simulink model "sm_3d_printer"  (R2022a)
settings: Solver=FixedStepAuto  StartTime=0.0  StopTime=inf  FixedStep=0.005  RelTol=1e-3
model workspace: external: MATLAB File sm_3d_printer_parameters.m (data not in the file)
undefined symbols (not defined in the file): smiData, X, Y, Z
libraries: sm_lib x33, fl_lib x15, nesl_utility x10, ee_lib x3, slpidlib x3
(part 1 of 3)
settings Model: PacingRate=0.250000  Creator=The MathWorks, Inc.  LastModifiedBy=ale
settings SolverCC: AlgebraicLoopSolver=TrustRegion
settings DataIOCC: ReturnWorkspaceOutputs=off  SignalLoggingName=logsout_sm_3d_printer  ReturnWorkspaceOutputsName=tp3277b97d_6d31_4550_b739_ddfa201eda0b
settings DebuggingCC: UnconnectedInputMsg=warning  UnconnectedOutputMsg=warning  UnconnectedLineMsg=warning  SFMachineParentedDataDiag=warning
settings RTWCC: DLArmComputeVersion=19.05
settings SimscapeCC: SimscapeLogType=all  SimscapeLogSimulationStatistics=on  SimscapeLogName=simlog_sm_3d_printer  SimscapeLogLimitData=off  SimscapeLogDataHistory=6000
settings ExplorerConfigSet: InternalSimMechanicsExplorerSettings="<ExplorerConfiguration><canonicalview>default</canonicalview><AnimationSetting><BasePlaybackSpeed>1.0</BasePlaybackSpeed><PlaybackSpeedFactor>1.0</PlaybackSpeedFactor></AnimationSetting><TilePanel><TileInfo><Tiles Columns=\"2\" Count=\"3\" Rows=\"2\"><Column Weight=\"0.4991\"/><Column Weight=\"0.5009\"/><Row Weight=\"0.5\"/><Row Weight=\"0.5\"/><Tile Height=\"2\" Width=\"1\" X=\"0\" Y=\"0\"/><Tile Height=\"1\" Width=\"1\" X=\"1\" Y=\"0\"/><Tile Height=\"1\" Width=\"1\" X=\"1\" Y=\"1\"/></Tiles></TileInfo><SceneInfo><SceneViewer><BGColor><R>1</R><G>1</G><B>1</B></BGColor><Camera><DoPerspective>off</DoPerspective><Position><X>0.517183646619549187</X><Y>-0.517183616511187494</Y><Z>0.756683602090616692</Z></Position><Center><X>-0.0601666225700767041</X><Y>0.0601666526784384315</Y><Z>0.179333332900990905</Z></Center><Up><X>-0.408248290463863073</X><Y>0.408248290463863073</Y><Z>0.816496580927726145</Z></Up><ViewLimDist>1</ViewLimDist><YLim>0.950683694503029364</YLim><XLim>0.650749683842918647</XLim></Camera></SceneViewer><SceneViewer><BGColor><R>1</R><G>1</G><B>1</B></BGColor><Camera><DoPerspective>off</DoPerspective><Position><X>-0.0490736034624795273</X><Y>-0.0707121472427751085</Y><Z>1.81681125048728176</Z></Position><Center><X>-0.0490736034624795273</X><Y>-0.0707121472427751085</Y><Z>0.388900037674711374</Z></Center><Up><X>0</X><Y>1</Y><Z>-0</Z></Up><ViewLimDist>1</ViewLimDist><YLim>0.613605105866690814</YLim><XLim>0.865431478794638998</XLim></Camera></SceneViewer><SceneViewer><BGColor><R>1</R><G>1</G><B>1</B></BGColor><Camera><DoPerspective>off</DoPerspective><Position><X>-0.0653022372858333144</X><Y>-1.68343497325259128</Y><Z>0.329149100724004773</Z></Position><Center><X>-0.0653022372858333144</X><Y>-0.0588999497118882775</Y><Z>0.329149100724004773</Z></Center><Up><X>0</X><Y>-0</Y><Z>1</Z></Up><ViewLimDist>1</ViewLimDist><YLim>0.614884320576226218</YLim><XLim>0.867235689136411469</XLim></Camera></SceneViewer></SceneInfo></TilePanel><MechEditorPanel><Cameras/><GfxPanelCameraMap/><VideoCreator><PlaybackSpeedRatio>1.0</PlaybackSpeedRatio><FrameRate>30</FrameRate><VideoFormat>Motion JPEG AVI</VideoFormat><FrameSize>auto</FrameSize></VideoCreator></MechEditorPanel></ExplorerConfiguration>"

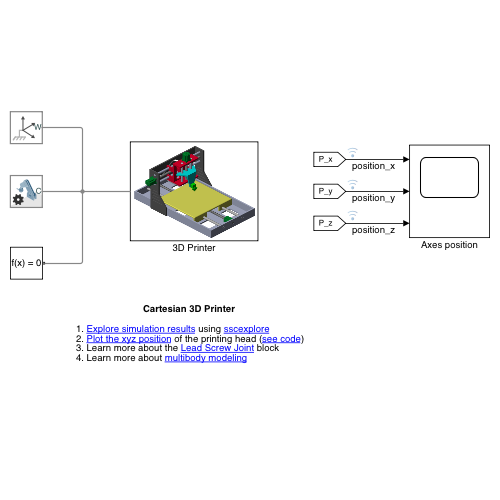
[thumbnail: Simulink's stored preview of the top-level diagram]
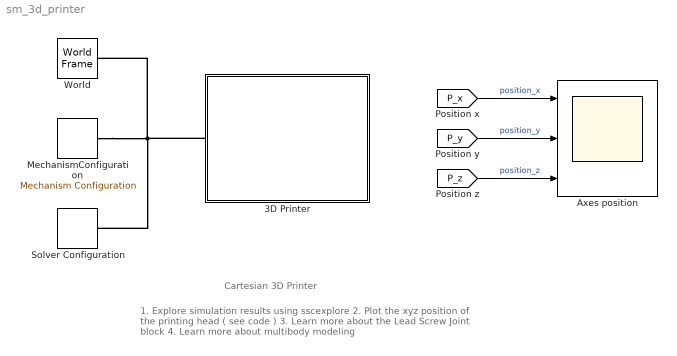
== system sm_3d_printer ==
  note: 1. Explore simulation results using sscexplore
      | 2. Plot the xyz position of the printing head ( see code )
      | 3. Learn more about the Lead Screw Joint block
      | 4. Learn more about multibody modeling
  note: Cartesian 3D Printer
  3D Printer : Subsystem
      mask Display: image('Printer_mask_empty.png');
  Axes position : Scope  NumInputPorts=3
  MechanismConfiguration : sm_lib/Utilities/Mechanism Configuration  UniformGravity=Constant  GravityVector=[0 0 -9.80665]  GravityUnits=m/s^2  LinearizationDelta=0.001  JointModeTransitionNonlinearIterations=2
  Solver Configuration : nesl_utility/Solver Configuration  PhysicalDomain=network_engine_domain  SubClassName=solver  LeftPortType=input  RightPortType=generic  Tones=[]  Harmonics=[]  SimulateNoise=off  Profile=off  UseLocalSampling=off  EnableSwitchedLinearOptims=on  FrequencyDomain=off  UseCCode=off  RelTol=0.001  AbsTol=1e-06  MinStep=1e-09  ToWorkspace=off  RevertToSquareIcSolve=off  NumHomotopyIterations=100  PhasorMode=off  PhasorModeNumHarmonics=1  IndexReductionMethod=DerivativeReplacement  DoDC=off  ResidualTolerance=1e-09  UseLocalSolver=off  LocalSolverChoice=NE_BACKWARD_EULER_ADVANCER  LocalSolverSampleTime=0.001  DoFixedCost=off  MaxNonlinIter=3  MaxModeIter=2  ComputeImpulses=off  ImpulseIterations=1  LinearAlgebra=auto  LinearAlgebraNumThread=0  EquationFormulation=NE_TIME_EF  DelaysMemoryBudget=1024  AutomaticFiltering=on  FilteringTimeConstant=0.001  PartitionStorageMethod=AS_NEEDED  PartitionMemoryBudget=1024  PartitionMethod=ROBUST
      settings: SourceProductBaseCode=SS,PW,VE
  World : sm_lib/Frames and Transforms/World Frame
  wires:
  [P_x] -> Axes position/1  "position_x"
  [P_y] -> Axes position/2  "position_y"
  [P_z] -> Axes position/3  "position_z"
  connections:
  MechanismConfiguration/RConn1 -- Solver Configuration/RConn1 -- 3D Printer/LConn1 -- World/RConn1

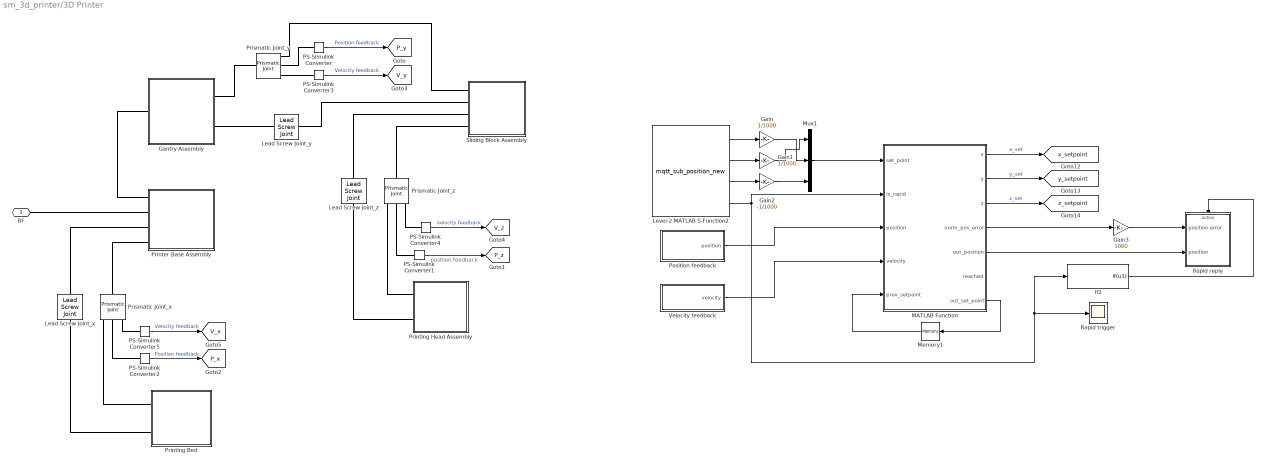
== system sm_3d_printer/3D Printer ==
  note: position feedback
  Gain : Gain  Gain=1/1000
  Gain1 : Gain  Gain=1/1000
  Gain2 : Gain  Gain=-1/1000
  Gain3 : Gain  Gain=1000
  Gantry Assembly : Subsystem  mask(Printer Gantry){}
      mask help:
      | This block models the gantry of the 3d printer. This block contains a linear actuator and a gantry. The linear actuator drives the motion of the sliding block along the y-axis.
      |
      | Port LB corresponds to the connection between the printer base and gantry assemblies. It is located at the top right corner on the bottom surface of the left leg of the gantry.
      |
      | Port BotH corresponds to the connection point to the bottom guide rail and is located at the central point of the bottom hole on the right leg of the gantry.
      |
      | Port LS corresponds to the lead screw connection and is located at the center of the right end of the lead screw.
      mask Display: image('Gantry_Assembly.png');
  If2 : If  IfExpression=u1  ShowElse=off
  Lead Screw Joint_x : sm_lib/Joints/Lead Screw Joint  JointMode=Normal  SenseConstraintForce=off  SenseConstraintForceX=off  SenseConstraintForceY=off  SenseConstraintForceZ=off  SenseConstraintTorque=off  SenseConstraintTorqueX=off  SenseConstraintTorqueY=off  SenseConstraintTorqueZ=off  SenseTotalForce=off  SenseTotalForceX=off  SenseTotalForceY=off  SenseTotalForceZ=off  SenseTotalTorque=off  SenseTotalTorqueX=off  SenseTotalTorqueY=off  SenseTotalTorqueZ=off  CompositeWrenchDir=FollowerOnBase  CompositeWrenchFrame=BaseFrame  Direction=RightHand  Lead=1.0  LeadUnits=cm/rev  SenseRotationPosition=off  SenseRotationVelocity=off  SenseRotationAcceleration=off  SenseTranslationPosition=off  SenseTranslationVelocity=off  SenseTranslationAcceleration=off  PositionTargetSpecify=off  PositionTargetPriority=High  PositionTargetRotationBased=off  PositionTargetRotationValue=0  PositionTargetRotationValueUnits=deg  PositionTargetTranslationValue=0.03  PositionTargetTranslationValueUnits=m  VelocityTargetSpecify=off  VelocityTargetPriority=High  VelocityTargetRotationBased=off  VelocityTargetRotationValue=0  VelocityTargetRotationValueUnits=deg/s  VelocityTargetTranslationValue=0  VelocityTargetTranslationValueUnits=m/s
      settings: SourceProductBaseCode=MS
  Lead Screw Joint_y : sm_lib/Joints/Lead Screw Joint  JointMode=Normal  SenseConstraintForce=off  SenseConstraintForceX=off  SenseConstraintForceY=off  SenseConstraintForceZ=off  SenseConstraintTorque=off  SenseConstraintTorqueX=off  SenseConstraintTorqueY=off  SenseConstraintTorqueZ=off  SenseTotalForce=off  SenseTotalForceX=off  SenseTotalForceY=off  SenseTotalForceZ=off  SenseTotalTorque=off  SenseTotalTorqueX=off  SenseTotalTorqueY=off  SenseTotalTorqueZ=off  CompositeWrenchDir=FollowerOnBase  CompositeWrenchFrame=BaseFrame  Direction=RightHand  Lead=1  LeadUnits=cm/rev  SenseRotationPosition=off  SenseRotationVelocity=off  SenseRotationAcceleration=off  SenseTranslationPosition=off  SenseTranslationVelocity=off  SenseTranslationAcceleration=off  PositionTargetSpecify=off  PositionTargetPriority=High  PositionTargetRotationBased=off  PositionTargetRotationValue=0  PositionTargetRotationValueUnits=deg  PositionTargetTranslationValue=0.398  PositionTargetTranslationValueUnits=m  VelocityTargetSpecify=off  VelocityTargetPriority=High  VelocityTargetRotationBased=on  VelocityTargetRotationValue=120  VelocityTargetRotationValueUnits=deg/s  VelocityTargetTranslationValue=0  VelocityTargetTranslationValueUnits=m/s
      settings: SourceProductBaseCode=MS
  Lead Screw Joint_z : sm_lib/Joints/Lead Screw Joint  JointMode=Normal  SenseConstraintForce=off  SenseConstraintForceX=off  SenseConstraintForceY=off  SenseConstraintForceZ=off  SenseConstraintTorque=off  SenseConstraintTorqueX=off  SenseConstraintTorqueY=off  SenseConstraintTorqueZ=off  SenseTotalForce=off  SenseTotalForceX=off  SenseTotalForceY=off  SenseTotalForceZ=off  SenseTotalTorque=off  SenseTotalTorqueX=off  SenseTotalTorqueY=off  SenseTotalTorqueZ=off  CompositeWrenchDir=FollowerOnBase  CompositeWrenchFrame=BaseFrame  Direction=RightHand  Lead=1.0  LeadUnits=cm/rev  SenseRotationPosition=off  SenseRotationVelocity=off  SenseRotationAcceleration=off  SenseTranslationPosition=off  SenseTranslationVelocity=off  SenseTranslationAcceleration=off  PositionTargetSpecify=off  PositionTargetPriority=High  PositionTargetRotationBased=off  PositionTargetRotationValue=0  PositionTargetRotationValueUnits=deg  PositionTargetTranslationValue=0.398  PositionTargetTranslationValueUnits=m  VelocityTargetSpecify=off  VelocityTargetPriority=High  VelocityTargetRotationBased=on  VelocityTargetRotationValue=120  VelocityTargetRotationValueUnits=deg/s  VelocityTargetTranslationValue=0  VelocityTargetTranslationValueUnits=m/s
      settings: SourceProductBaseCode=MS
  Level-2 MATLAB S-Function2 : M-S-Function  FunctionName=mqtt_sub_position_new
  MATLAB Function : MATLAB Function  TreatAsAtomicUnit=on
  Memory1 : Memory  InitialCondition=[0;0;0]  InheritSampleTime=on  LinearizeAsDelay=on
  Mux1 : Mux  Inputs=3
  PS-Simulink Converter : nesl_utility/PS-Simulink Converter  PhysicalDomain=network_engine_domain  SubClassName=ps_output  LeftPortType=input  RightPortType=output  PseudoPeriodic=off  Frequencies=[]  VectorFormat=1-D array  Unit=m  AffineConversion=off
      settings: SourceProductBaseCode=SS,PW,VE
  PS-Simulink Converter1 : nesl_utility/PS-Simulink Converter  PhysicalDomain=network_engine_domain  SubClassName=ps_output  LeftPortType=input  RightPortType=output  PseudoPeriodic=off  Frequencies=[]  VectorFormat=1-D array  Unit=m  AffineConversion=off
      settings: SourceProductBaseCode=SS,PW,VE
  PS-Simulink Converter2 : nesl_utility/PS-Simulink Converter  PhysicalDomain=network_engine_domain  SubClassName=ps_output  LeftPortType=input  RightPortType=output  PseudoPeriodic=off  Frequencies=[]  VectorFormat=1-D array  Unit=m  AffineConversion=off
      settings: SourceProductBaseCode=SS,PW,VE
  PS-Simulink Converter3 : nesl_utility/PS-Simulink Converter  PhysicalDomain=network_engine_domain  SubClassName=ps_output  LeftPortType=input  RightPortType=output  PseudoPeriodic=off  Frequencies=[]  VectorFormat=1-D array  Unit=m/s  AffineConversion=off
      settings: SourceProductBaseCode=SS,PW,VE
  PS-Simulink Converter4 : nesl_utility/PS-Simulink Converter  PhysicalDomain=network_engine_domain  SubClassName=ps_output  LeftPortType=input  RightPortType=output  PseudoPeriodic=off  Frequencies=[]  VectorFormat=1-D array  Unit=m/s  AffineConversion=off
      settings: SourceProductBaseCode=SS,PW,VE
  PS-Simulink Converter5 : nesl_utility/PS-Simulink Converter  PhysicalDomain=network_engine_domain  SubClassName=ps_output  LeftPortType=input  RightPortType=output  PseudoPeriodic=off  Frequencies=[]  VectorFormat=1-D array  Unit=m/s  AffineConversion=off
      settings: SourceProductBaseCode=SS,PW,VE
  Position feedback : Subsystem
  Printer Base Assembly : Subsystem  mask(Printer Base Assembly){}
      mask help:
      | This block models the base assembly of the 3d printer. This block contains one linear actuator and the base of the printer. The linear actuator drives the motion of the printing bed along the x-axis.
      |
      | Port ML corresponds to the connection between the printer base and gantry assemblies. It is located at the middle point of the left edge of the base.
      |
      | Port BF cooresponds to the connection between the world frame and the base frame of the printer base. It is located at the center of the bottom surface of the printer base.
      |
      | Port GR corresponds to the connection point to the left guide rail and is located at the center of one end of the guide rail.
      |
      | Port LS corresponds to the lead screw connection and is located at the central point of the lead screw.
      mask Display: image('Base_Assembly.png');
  "Printing Bed " : Subsystem  mask(Printing Bed){}
      mask help:
      | This block models the printing bed of the 3d printer.
      |
      | Port LH corresponds to the connection point to the left guide rail and is located at the central point of the left hole on the rear face of the printing bed.
      |
      | Port CH corresponds to the lead screw connection and is located at the central point of the hole located at the central block of the printing bed.
      mask Display: image('$imagefile'); % Use "Edit Image" on toolstrip to change.
  Printing Head Assembly : Subsystem  mask(Printing Head Assembly){}
      mask help:
      | This block models the printing head assembly of the 3d printer. This block contains one printing head and its bracket.
      |
      | Port RH corresponds to the connection point to the right guide rail and is located at the central point of the right hole on the bracket.
      |
      | Port LS corresponds to the lead screw connection and is located at the central point of the middle hole on the bracket.
      mask Display: image('Printing_Head_Assembly.png');
  Prismatic Joint_x : sm_lib/Joints/Prismatic Joint  JointMode=Normal  SenseConstraintForce=off  SenseConstraintForceX=off  SenseConstraintForceY=off  SenseConstraintForceZ=off  SenseConstraintTorque=off  SenseConstraintTorqueX=off  SenseConstraintTorqueY=off  SenseConstraintTorqueZ=off  SenseTotalForce=off  SenseTotalForceX=off  SenseTotalForceY=off  SenseTotalForceZ=off  SenseTotalTorque=off  SenseTotalTorqueX=off  SenseTotalTorqueY=off  SenseTotalTorqueZ=off  CompositeWrenchDir=FollowerOnBase  CompositeWrenchFrame=BaseFrame  EquilibriumPosition=0  EquilibriumPositionUnits=m  SpringStiffness=0  SpringStiffnessUnits=N/m  DampingCoefficient=0  DampingCoefficientUnits=N/(m/s)  TorqueActuationMode=NoTorque  MotionActuationMode=ComputedMotion  SensePosition=on  SenseVelocity=on  SenseAcceleration=off  SenseTorqueForce=off  SenseLowerLimitTorqueForce=off  SenseUpperLimitTorqueForce=off  LowerLimitSpecify=off  LowerLimitBound=-1  LowerLimitBoundUnits=m  LowerLimitStiffness=1e6  LowerLimitStiffnessUnits=N/m  LowerLimitDamping=1e3  LowerLimitDampingUnits=N/(m/s)  LowerLimitTransitionRegionWidth=1e-4  LowerLimitTransitionRegionWidthUnits=m  UpperLimitSpecify=off  UpperLimitBound=1  UpperLimitBoundUnits=m  UpperLimitStiffness=1e6  UpperLimitStiffnessUnits=N/m  UpperLimitDamping=1e3  UpperLimitDampingUnits=N/(m/s)  UpperLimitTransitionRegionWidth=1e-4  UpperLimitTransitionRegionWidthUnits=m  PositionTargetSpecify=off  PositionTargetPriority=High  PositionTargetValue=smiData.offset(2).value  PositionTargetValueUnits=m  VelocityTargetSpecify=off  VelocityTargetPriority=High  VelocityTargetValue=0  VelocityTargetValueUnits=m/s
  Prismatic Joint_y : sm_lib/Joints/Prismatic Joint  JointMode=Normal  SenseConstraintForce=off  SenseConstraintForceX=off  SenseConstraintForceY=off  SenseConstraintForceZ=off  SenseConstraintTorque=off  SenseConstraintTorqueX=off  SenseConstraintTorqueY=off  SenseConstraintTorqueZ=off  SenseTotalForce=off  SenseTotalForceX=off  SenseTotalForceY=off  SenseTotalForceZ=off  SenseTotalTorque=off  SenseTotalTorqueX=off  SenseTotalTorqueY=off  SenseTotalTorqueZ=off  CompositeWrenchDir=FollowerOnBase  CompositeWrenchFrame=BaseFrame  EquilibriumPosition=0  EquilibriumPositionUnits=m  SpringStiffness=0  SpringStiffnessUnits=N/m  DampingCoefficient=0  DampingCoefficientUnits=N/(m/s)  TorqueActuationMode=NoTorque  MotionActuationMode=ComputedMotion  SensePosition=on  SenseVelocity=on  SenseAcceleration=off  SenseTorqueForce=off  SenseLowerLimitTorqueForce=off  SenseUpperLimitTorqueForce=off  LowerLimitSpecify=off  LowerLimitBound=-1  LowerLimitBoundUnits=m  LowerLimitStiffness=1e6  LowerLimitStiffnessUnits=N/m  LowerLimitDamping=1e3  LowerLimitDampingUnits=N/(m/s)  LowerLimitTransitionRegionWidth=1e-4  LowerLimitTransitionRegionWidthUnits=m  UpperLimitSpecify=off  UpperLimitBound=1  UpperLimitBoundUnits=m  UpperLimitStiffness=1e6  UpperLimitStiffnessUnits=N/m  UpperLimitDamping=1e3  UpperLimitDampingUnits=N/(m/s)  UpperLimitTransitionRegionWidth=1e-4  UpperLimitTransitionRegionWidthUnits=m  PositionTargetSpecify=off  PositionTargetPriority=High  PositionTargetValue=smiData.offset(2).value  PositionTargetValueUnits=m  VelocityTargetSpecify=off  VelocityTargetPriority=High  VelocityTargetValue=0  VelocityTargetValueUnits=m/s
  Prismatic Joint_z : sm_lib/Joints/Prismatic Joint  JointMode=Normal  SenseConstraintForce=off  SenseConstraintForceX=off  SenseConstraintForceY=off  SenseConstraintForceZ=off  SenseConstraintTorque=off  SenseConstraintTorqueX=off  SenseConstraintTorqueY=off  SenseConstraintTorqueZ=off  SenseTotalForce=off  SenseTotalForceX=off  SenseTotalForceY=off  SenseTotalForceZ=off  SenseTotalTorque=off  SenseTotalTorqueX=off  SenseTotalTorqueY=off  SenseTotalTorqueZ=off  CompositeWrenchDir=FollowerOnBase  CompositeWrenchFrame=BaseFrame  EquilibriumPosition=0  EquilibriumPositionUnits=m  SpringStiffness=0  SpringStiffnessUnits=N/m  DampingCoefficient=0  DampingCoefficientUnits=N/(m/s)  TorqueActuationMode=NoTorque  MotionActuationMode=ComputedMotion  SensePosition=on  SenseVelocity=on  SenseAcceleration=off  SenseTorqueForce=off  SenseLowerLimitTorqueForce=off  SenseUpperLimitTorqueForce=off  LowerLimitSpecify=off  LowerLimitBound=-1  LowerLimitBoundUnits=m  LowerLimitStiffness=1e6  LowerLimitStiffnessUnits=N/m  LowerLimitDamping=1e3  LowerLimitDampingUnits=N/(m/s)  LowerLimitTransitionRegionWidth=1e-4  LowerLimitTransitionRegionWidthUnits=m  UpperLimitSpecify=off  UpperLimitBound=1  UpperLimitBoundUnits=m  UpperLimitStiffness=1e6  UpperLimitStiffnessUnits=N/m  UpperLimitDamping=1e3  UpperLimitDampingUnits=N/(m/s)  UpperLimitTransitionRegionWidth=1e-4  UpperLimitTransitionRegionWidthUnits=m  PositionTargetSpecify=off  PositionTargetPriority=High  PositionTargetValue=smiData.offset(2).value  PositionTargetValueUnits=m  VelocityTargetSpecify=off  VelocityTargetPriority=High  VelocityTargetValue=0  VelocityTargetValueUnits=m/s
  Rapid reply : Subsystem  TreatAsAtomicUnit=on
  Rapid trigger : Scope
  Sliding Block Assembly : Subsystem  mask(Sliding Block Assembly){}
      mask help:
      | This block models the sliding block assembly of the 3d printer. This block contains a linear actuator and a sliding block. The linear actuator drives the motion of the printing head along the z-axis.
      |
      | Port RBH corresponds to the connection point to the bottom guide rail and is located at the central point of the hole on the right side of the sliding block.
      |
      | Port HS corresponds to the lead screw connection and is located at the central point of the hole located at the central block of the sliding block.
      |
      | Port VS corresponds to the lead screw connection and is located at the central point of the hole located at the top surface of the sliding block.
      |
      | Port RB corresponds to the connection point to the right guide rail and is located at the central point of the right hole on the bottom surface of the sliding block.
      mask Display: image('Sliding_Block.png');
  Velocity feedback : Subsystem
  "BF " : PMIOPort  Side=Left
  tag scope: P_x=global, P_y=global, P_z=global, V_x=global, V_y=global, V_z=global, x_setpoint=global, y_setpoint=global, z_setpoint=global
  wires:
  PS-Simulink Converter1/1 -> [P_z]
  PS-Simulink Converter/1 -> [P_y]  "Position feedback"
  PS-Simulink Converter2/1 -> [P_x]  "Position feedback"
  PS-Simulink Converter3/1 -> [V_y]  "Velocity feedback"
  PS-Simulink Converter4/1 -> [V_z]  "velocity feedback"
  PS-Simulink Converter5/1 -> [V_x]  "Velocity feedback"
  MATLAB Function/7(out_set_point) -> Memory1/1
  Mux1/1 -> MATLAB Function/1(set_point)
  MATLAB Function/3(z) -> [z_setpoint]  "z_set"
  Level-2 MATLAB S-Function2/4 -> Rapid trigger/1, If2/1, MATLAB Function/2(is_rapid)
  Velocity feedback/1(velocity) -> MATLAB Function/4(velocity)
  MATLAB Function/1(x) -> [x_setpoint]  "x_set"
  MATLAB Function/2(y) -> [y_setpoint]  "y_set"
  Position feedback/1(position) -> MATLAB Function/3(position)
  Memory1/1 -> MATLAB Function/5(prev_setpoint)
  Level-2 MATLAB S-Function2/1 -> Gain/1
  Level-2 MATLAB S-Function2/2 -> Gain1/1
  Level-2 MATLAB S-Function2/3 -> Gain2/1
  MATLAB Function/4(norm_pos_error) -> Gain3/1
  If2/1 -> Rapid reply/Action
  MATLAB Function/5(out_position) -> Rapid reply/2(position)
  Gain/1 -> Mux1/2
  Gain1/1 -> Mux1/1
  Gain2/1 -> Mux1/3
  Gain3/1 -> Rapid reply/1(position error)
  connections:
  Printer Base Assembly/LConn2 -- "BF "/RConn1
  Prismatic Joint_y/LConn1 -- Gantry Assembly/RConn1
  Printing Head Assembly/LConn1 -- Prismatic Joint_z/RConn1
  Sliding Block Assembly/LConn2 -- Lead Screw Joint_y/RConn1
  Lead Screw Joint_z/RConn1 -- Printing Head Assembly/LConn2
  Prismatic Joint_y/RConn1 -- Sliding Block Assembly/LConn1
  Printer Base Assembly/LConn1 -- Gantry Assembly/LConn1
  PS-Simulink Converter1/LConn1 -- Prismatic Joint_z/RConn2
  Lead Screw Joint_y/LConn1 -- Gantry Assembly/RConn2
  Sliding Block Assembly/LConn3 -- Lead Screw Joint_z/LConn1
  Lead Screw Joint_x/LConn1 -- Printer Base Assembly/LConn3
  Lead Screw Joint_x/RConn1 -- "Printing Bed "/RConn2
  Prismatic Joint_y/RConn2 -- PS-Simulink Converter/LConn1
  Prismatic Joint_y/RConn3 -- PS-Simulink Converter3/LConn1
  Sliding Block Assembly/LConn4 -- Prismatic Joint_z/LConn1
  Prismatic Joint_z/RConn3 -- PS-Simulink Converter4/LConn1
  Prismatic Joint_x/LConn1 -- Printer Base Assembly/LConn4
  Prismatic Joint_x/RConn1 -- "Printing Bed "/RConn1
  Prismatic Joint_x/RConn2 -- PS-Simulink Converter2/LConn1
  Prismatic Joint_x/RConn3 -- PS-Simulink Converter5/LConn1

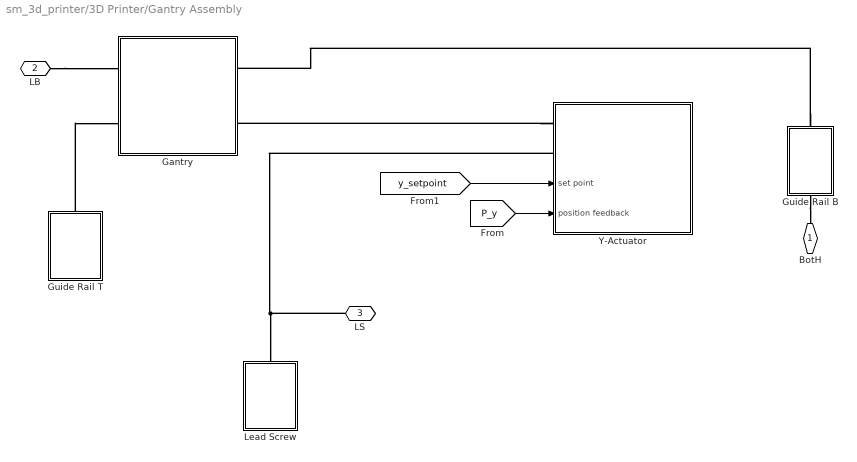
== system sm_3d_printer/3D Printer/Gantry Assembly ==
  Gantry : Subsystem  mask(Gantry){}
      mask help:
      | This block models the gantry of the 3d printer.
      |
      | Port LB corresponds to the connection between the printer base and gantry assemblies. It is located at the top right corner on the bottom surface of the left leg of the gantry.
      |
      | Port TopH and  BotH correspond to the connection points to the guide rails and are located at the central points of the holes on the right leg of the gantry.
      |
      | Port MidH corresponds to the lead screw connection and is located at the central point of the middle hole on the right leg of the gantry.
      mask Display: image('Gantry.png');
  Guide Rail B : Subsystem  mask(Guide Rail){}
      mask help:
      | This block models a guide rail of the linear actuator.
      |
      | The ports L and R correspond to the central points of the two end faces.
      mask Display: image('Bar.png');
  Guide Rail T : Subsystem  mask(Guide Rail){}
      mask help:
      | This block models a guide rail of the linear actuator.
      |
      | The ports L and R correspond to the central points of the two end faces.
      mask Display: image('Bar.png');
  Lead Screw : Subsystem  mask(Lead Screw){}
      mask help:
      | This block models the lead screw of the linear actuator.
      |
      | The ports L and R correspond to the central points of the two end faces.
      mask Display: image('Screw.png');
  Y-Actuator : Subsystem  mask(Printing Head Assembly){}
      mask help:
      | This block models the printing head assembly of the 3d printer. This block contains one printing head and its bracket.
      |
      | Port RH corresponds to the connection point to the right guide rail and is located at the central point of the right hole on the bracket.
      |
      | Port LS corresponds to the lead screw connection and is located at the central point of the middle hole on the bracket.
      settings: PortSchema="{\"entries\":[{\"content\":{\"sides\":[{\"content\":{\"connectorIds\":[\"LConn1\",\"LConn2\",\"In1\",\"In2\"]},\"type\":\"ConnectorPlacement.EquallySpacedRectSide\",\"uuid\":\"22a72145-70fe-4c07-a355-17651bab5534\"},{\"content\":{\"connectorIds\":[],\"side\":\"RIGHT\"},\"type\":\"ConnectorPlacement.EquallySpacedRectSide\",\"uuid\":\"e15c401c-ae36-45b1-bf72-5294abc9e452\"},{\"content\":{\"connectorIds\":[],\"side\":\"TOP\"},\"type\":\"ConnectorPlacement.EquallySpacedRectSide\",\"uuid\":\"2bd32be4-c9a2-44f1-9e48-22d0cf521a2c\"}]},\"type\":\"ConnectorPlacement.EquallySpacedConnector\",\"uuid\":\"b7677459-9517-441c-aa48-c4152952097c\"}],\"packageUris\":[\"http://schema.mathworks.com/mf0/Connector/R2020b\"],\"version\":\"1.0\"}"
      mask Display: image('Stepper_motor.png');
  BotH : PMIOPort  Side=Right
  LB : PMIOPort  Port=2  Side=Left
  "LS " : PMIOPort  Port=3  Side=Right
  wires:
  [P_y] -> Y-Actuator/2(position feedback)
  [y_setpoint] -> Y-Actuator/1(set point)
  connections:
  Guide Rail B/LConn1 -- Gantry/RConn1
  Guide Rail T/LConn1 -- Gantry/LConn2
  LB/RConn1 -- Gantry/LConn1
  "LS "/RConn1 -- Y-Actuator/LConn2 -- Lead Screw/LConn1
  Guide Rail B/RConn1 -- BotH/RConn1
  Y-Actuator/LConn1 -- Gantry/RConn2

== system sm_3d_printer/3D Printer/Position feedback ==
  Mux1 : Mux  Inputs=3
  position : Outport
  wires:
  Mux1/1 -> position/1
  [P_y] -> Mux1/2
  [P_z] -> Mux1/3
  [P_x] -> Mux1/1

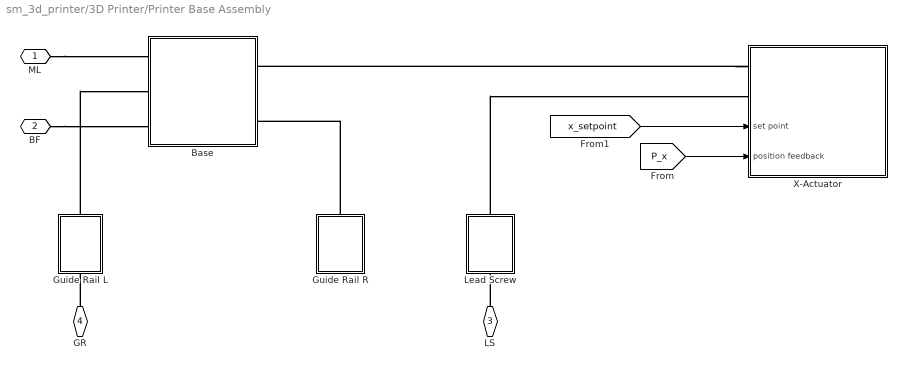
== system sm_3d_printer/3D Printer/Printer Base Assembly ==
  Base : Subsystem  mask(Base){}
      mask help:
      | This block models the base of the 3D printer.
      |
      | Port ML corresponds to the connection between the printer base and gantry assemblies. It locates at the middle point of the left edge of the base.
      | Port Base is the base frame of the printer base and is located at the center of the bottom surface of the base.
      | Port MH corresponds to the lead screw connection and is located at the central point of the hole located at the center of the front surface of the base.
      | Port LH and RH correspond to the connection points to the guide rails and are located at the central point of the holes on the front surface of the base.
      mask Display: image('Base.png'); % Use "Edit Image" on toolstrip to change.
  Guide Rail L : Subsystem  mask(Guide Rail){}
      mask help:
      | This block models a guide rail of the linear actuator.
      |
      | The ports L and R correspond to the central points of the two end faces.
      mask Display: image('Bar.png'); % Use "Edit Image" on toolstrip to change.
  Guide Rail R : Subsystem  mask(Guide Rail){}
      mask help:
      | This block models a guide rail of the linear actuator.
      |
      | The ports L and R correspond to the central points of the two end faces.
      mask Display: image('Bar.png'); % Use "Edit Image" on toolstrip to change.
  Lead Screw : Subsystem  mask(Lead Screw){}
      mask help:
      | This block models the lead screw of the linear actuator.
      |
      | Ports L corresponds to the center of the left end.
      | Port CP corresponds to the central point of the lead screw.
      mask Display: image('Screw.png'); % Use "Edit Image" on toolstrip to change.
  X-Actuator : Subsystem  mask(Printing Head Assembly){}
      mask help:
      | This block models the printing head assembly of the 3d printer. This block contains one printing head and its bracket.
      |
      | Port RH corresponds to the connection point to the right guide rail and is located at the central point of the right hole on the bracket.
      |
      | Port LS corresponds to the lead screw connection and is located at the central point of the middle hole on the bracket.
      settings: PortSchema="{\"entries\":[{\"content\":{\"sides\":[{\"content\":{\"connectorIds\":[\"LConn1\",\"LConn2\",\"In1\",\"In2\"]},\"type\":\"ConnectorPlacement.EquallySpacedRectSide\",\"uuid\":\"22a72145-70fe-4c07-a355-17651bab5534\"},{\"content\":{\"connectorIds\":[],\"side\":\"RIGHT\"},\"type\":\"ConnectorPlacement.EquallySpacedRectSide\",\"uuid\":\"e15c401c-ae36-45b1-bf72-5294abc9e452\"},{\"content\":{\"connectorIds\":[],\"side\":\"TOP\"},\"type\":\"ConnectorPlacement.EquallySpacedRectSide\",\"uuid\":\"2bd32be4-c9a2-44f1-9e48-22d0cf521a2c\"}]},\"type\":\"ConnectorPlacement.EquallySpacedConnector\",\"uuid\":\"b7677459-9517-441c-aa48-c4152952097c\"}],\"packageUris\":[\"http://schema.mathworks.com/mf0/Connector/R2020b\"],\"version\":\"1.0\"}"
      mask Display: image('Stepper_motor.png');
  ML : PMIOPort  Side=Left
  "BF " : PMIOPort  Port=2  Side=Left
  LS : PMIOPort  Port=3  Side=Left
  GR : PMIOPort  Port=4  Side=Left
  wires:
  [P_x] -> X-Actuator/2(position feedback)
  [x_setpoint] -> X-Actuator/1(set point)
  connections:
  Guide Rail L/LConn1 -- Base/LConn2
  Guide Rail R/RConn1 -- Base/RConn2
  ML/RConn1 -- Base/LConn1
  "BF "/RConn1 -- Base/LConn3
  GR/RConn1 -- Guide Rail L/RConn1
  LS/RConn1 -- Lead Screw/LConn1
  X-Actuator/LConn1 -- Base/RConn1
  Lead Screw/RConn1 -- X-Actuator/LConn2

== system sm_3d_printer/3D Printer/Printing Bed  ==
  Offset_x : sm_lib/Frames and Transforms/Rigid Transform  TranslationMethod=StandardAxis  TranslationStandardOffset=smiData.offset(1).value  TranslationLengthUnit=m  TranslationStandardAxis=+Z  TranslationCartesianOffset=[0 0 0]  TranslationROffset=0  TranslationROffsetUnits=m  TranslationZOffset=0  TranslationZOffsetUnits=m  TranslationThetaOffset=0  TranslationThetaOffsetUnits=deg  RotationMethod=None  RotationAngleUnits=deg  RotationStandardAxis=+Z  RotationAngle=0.0  RotationArbitraryAxis=[0 0 1]  FollAlignAxisA=+X  BaseAlignAxisA=+Y  FollAlignAxisB=+Y  BaseAlignAxisB=+Z  RotationSequenceAxes=FollowerAxes  RotationSequence=XYX  RotationSequenceAngles=[0 0 0]  RotationSequenceAnglesUnits=deg  RotationMatrix=[1 0 0; 0 1 0; 0 0 1]
  Printing Bed : sm_lib/Body Elements/File Solid  ExtGeomFileName=Printing_Bed.STEP  UnitType=FromFile  ExtGeomFileUnits=m  StepReaderType=HEX  ExportConvexHullGeometry=off  InertiaType=Custom  Mass=smiData.Solid(7).mass  MassUnits=kg  CenterOfMass=smiData.Solid(7).CoM  CenterOfMassUnits=m  MomentsOfInertia=smiData.Solid(7).MoI  MomentsOfInertiaUnits=kg*m^2  ProductsOfInertia=smiData.Solid(7).PoI  ProductsOfInertiaUnits=kg*m^2  BasedOnType=Density  Density=550  DensityUnits=kg/m^3  DoExposeReferenceFrame=off  SerializedFrames=<Frames><Frame><Id>Frame1</Id><Value><Name>LH</Name><Origin><Source>GeometricFeature</Source><FeatureName>circular curve 8</FeatureName></Origin><PrimaryAxis><DefinedDirection>-X</DefinedDirection><Source>ReferenceFrame</Source><SourceDirection>-Z</SourceDirection><FeatureName></FeatureName></PrimaryAxis><SecondaryAxis><DefinedDirection>+Y</DefinedDirection><Source>ReferenceFrame</Source><SourceDirection>-X</SourceDirection><FeatureName></FeatureName></SecondaryAxis></Value></Frame><Frame><Id>Frame2</Id><Value><Name>CH</Name><Origin><Source>GeometricFeature</Source><FeatureName>circular curve 18</FeatureName></Origin><PrimaryAxis><DefinedDirection>+X</DefinedDirection><Source>ReferenceFrame</Source><SourceDirection>+Z</SourceDirection><FeatureName></FeatureName></PrimaryAxis><SecondaryAxis><DefinedDirection>-Y</DefinedDirection><Source>ReferenceFrame</Source><SourceDirection>+X</SourceDirection><FeatureName></FeatureName></SecondaryAxis></Value></Frame><Frame><Id>Frame5</Id><Value><Name>LetterLocationF</Name><Origin><Source>GeometricFeature</Source><FeatureName>point 184</FeatureName></Origin><PrimaryAxis><DefinedDirection>+Z</DefinedDirection><Source>ReferenceFrame</Source><SourceDirection>+Z</SourceDirection><FeatureName></FeatureName></PrimaryAxis><SecondaryAxis><DefinedDirection>+X</DefinedDirection><Source>ReferenceFrame</Source><SourceDirection>+X</SourceDirection><FeatureName></FeatureName></SecondaryAxis></Value></Frame></Frames>  GraphicType=FromGeometry  MarkerShape=Sphere  MarkerSize=10  GraphicVisPropType=SimpleVisualProperties  GraphicDiffuseColor=[1.0 1.0 0.4]  GraphicSpecularColor=[0.5 0.5 0.5 1.0]  GraphicAmbientColor=[0.15 0.15 0.15 1]  GraphicEmissiveColor=[0.0 0 0.0 1]  GraphicShininess=50  GraphicOpacity=smiData.Solid(7).opacity
  LH : PMIOPort  Side=Right
  "CH " : PMIOPort  Port=2  Side=Right
  connections:
  LH/RConn1 -- Offset_x/LConn1
  Printing Bed/RConn1 -- "CH "/RConn1
  Offset_x/RConn1 -- Printing Bed/LConn1

== system sm_3d_printer/3D Printer/Printing Head Assembly ==
  Bracket : Subsystem
      mask Display: image('Mount.png'); % Use "Edit Image" on toolstrip to change.
  Printing Head : Subsystem
      mask Display: image('Printing_Head.png'); % Use "Edit Image" on toolstrip to change.
  RH : PMIOPort  Side=Left
  "LS " : PMIOPort  Port=2  Side=Left
  connections:
  Printing Head/RConn1 -- Bracket/LConn3
  "LS "/RConn1 -- Bracket/LConn2
  Bracket/LConn1 -- RH/RConn1

== system sm_3d_printer/3D Printer/Rapid reply ==
  position error : Inport
  position : Inport  Port=2
  Action Port : ActionPort  ActionPortLabel=if(u1)
  Level-2 MATLAB S-Function3 : M-S-Function  FunctionName=mqtt_pub_rapid_new  Parameters=M
  wires:
  position error/1 -> Level-2 MATLAB S-Function3/1
  position/1 -> Level-2 MATLAB S-Function3/2

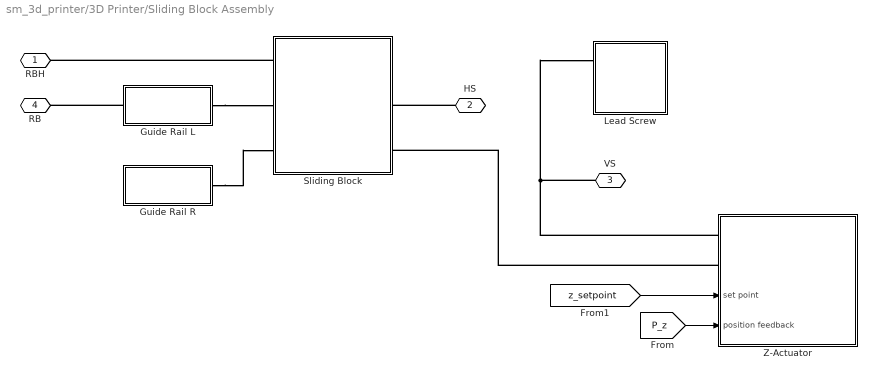
== system sm_3d_printer/3D Printer/Sliding Block Assembly ==
  "Guide Rail L " : Subsystem  mask(Guide Rail){}
      mask help:
      | This block models a guide rail of the linear actuator.
      |
      | The ports L and R correspond to the central points of the two end faces.
      mask Display: image('Bar.png');
  Guide Rail R : Subsystem  mask(Guide Rail){}
      mask help:
      | This block models a guide rail of the linear actuator.
      |
      | The ports L and R correspond to the central points of the two end faces.
      mask Display: image('Bar.png');
  Lead Screw : Subsystem  mask(Lead Screw){}
      mask help:
      | This block models the lead screw of the linear actuator.
      |
      | The ports L and R correspond to the central points of the two end faces.
      mask Display: image('Screw.png');
  Sliding Block : Subsystem
      mask Display: image('$imagefile'); % Use "Edit Image" on toolstrip to change.
  Z-Actuator : Subsystem  mask(Printing Head Assembly){}
      mask help:
      | This block models the printing head assembly of the 3d printer. This block contains one printing head and its bracket.
      |
      | Port RH corresponds to the connection point to the right guide rail and is located at the central point of the right hole on the bracket.
      |
      | Port LS corresponds to the lead screw connection and is located at the central point of the middle hole on the bracket.
      settings: PortSchema="{\"entries\":[{\"content\":{\"sides\":[{\"content\":{\"connectorIds\":[\"LConn1\",\"LConn2\",\"In1\",\"In2\"]},\"type\":\"ConnectorPlacement.EquallySpacedRectSide\",\"uuid\":\"22a72145-70fe-4c07-a355-17651bab5534\"},{\"content\":{\"connectorIds\":[],\"side\":\"RIGHT\"},\"type\":\"ConnectorPlacement.EquallySpacedRectSide\",\"uuid\":\"e15c401c-ae36-45b1-bf72-5294abc9e452\"},{\"content\":{\"connectorIds\":[],\"side\":\"TOP\"},\"type\":\"ConnectorPlacement.EquallySpacedRectSide\",\"uuid\":\"2bd32be4-c9a2-44f1-9e48-22d0cf521a2c\"}]},\"type\":\"ConnectorPlacement.EquallySpacedConnector\",\"uuid\":\"b7677459-9517-441c-aa48-c4152952097c\"}],\"packageUris\":[\"http://schema.mathworks.com/mf0/Connector/R2020b\"],\"version\":\"1.0\"}"
      mask Display: image('Stepper_motor.png');
  RBH : PMIOPort  Side=Left
  HS : PMIOPort  Port=2  Side=Left
  VS : PMIOPort  Port=3  Side=Left
  RB : PMIOPort  Port=4  Side=Left
  wires:
  [P_z] -> Z-Actuator/2(position feedback)
  [z_setpoint] -> Z-Actuator/1(set point)
  connections:
  Guide Rail R/RConn1 -- Sliding Block/RConn3
  "Guide Rail L "/RConn1 -- Sliding Block/RConn2
  Z-Actuator/LConn2 -- Sliding Block/LConn3
  VS/RConn1 -- Lead Screw/LConn1 -- Z-Actuator/LConn1
  Sliding Block/RConn1 -- RBH/RConn1
  HS/RConn1 -- Sliding Block/LConn2
  "Guide Rail L "/LConn1 -- RB/RConn1

== system sm_3d_printer/3D Printer/Velocity feedback ==
  Mux2 : Mux  Inputs=3
  velocity : Outport
  wires:
  Mux2/1 -> velocity/1
  [V_z] -> Mux2/3
  [V_y] -> Mux2/2
  [V_x] -> Mux2/1

== system sm_3d_printer/3D Printer/Gantry Assembly/Gantry ==
  Solid : sm_lib/Body Elements/File Solid  ExtGeomFileName=Gantry.STEP  UnitType=FromFile  ExtGeomFileUnits=m  StepReaderType=HEX  ExportConvexHullGeometry=off  InertiaType=Custom  Mass=smiData.Solid(10).mass  MassUnits=kg  CenterOfMass=smiData.Solid(10).CoM  CenterOfMassUnits=m  MomentsOfInertia=smiData.Solid(10).MoI  MomentsOfInertiaUnits=kg*m^2  ProductsOfInertia=smiData.Solid(10).PoI  ProductsOfInertiaUnits=kg*m^2  BasedOnType=DensityFromFile  Density=1000  DensityUnits=kg/m^3  DoExposeReferenceFrame=off  SerializedFrames=<Frames><Frame><Id>Frame1</Id><Value><Name>LB</Name><Origin><Source>GeometricFeature</Source><FeatureName>point 464</FeatureName></Origin><PrimaryAxis><DefinedDirection>+Z</DefinedDirection><Source>ReferenceFrame</Source><SourceDirection>+Z</SourceDirection><FeatureName></FeatureName></PrimaryAxis><SecondaryAxis><DefinedDirection>+X</DefinedDirection><Source>ReferenceFrame</Source><SourceDirection>+X</SourceDirection><FeatureName></FeatureName></SecondaryAxis></Value></Frame><Frame><Id>Frame2</Id><Value><Name>RB</Name><Origin><Source>GeometricFeature</Source><FeatureName>point 638</FeatureName></Origin><PrimaryAxis><DefinedDirection>+Z</DefinedDirection><Source>ReferenceFrame</Source><SourceDirection>+Z</SourceDirection><FeatureName></FeatureName></PrimaryAxis><SecondaryAxis><DefinedDirection>+X</DefinedDirection><Source>ReferenceFrame</Source><SourceDirection>+X</SourceDirection><FeatureName></FeatureName></SecondaryAxis></Value></Frame><Frame><Id>Frame3</Id><Value><Name>TopH</Name><Origin><Source>GeometricFeature</Source><FeatureName>circular curve 177</FeatureName></Origin><PrimaryAxis><DefinedDirection>+X</DefinedDirection><Source>ReferenceFrame</Source><SourceDirection>+Z</SourceDirection><FeatureName></FeatureName></PrimaryAxis><SecondaryAxis><DefinedDirection>+Y</DefinedDirection><Source>ReferenceFrame</Source><SourceDirection>+X</SourceDirection><FeatureName></FeatureName></SecondaryAxis></Value></Frame><Frame><Id>Frame4</Id><Value><Name>MidH</Name><Origin><Source>GeometricFeature</Source><FeatureName>circular curve 176</FeatureName></Origin><PrimaryAxis><DefinedDirection>+X</DefinedDirection><Source>ReferenceFrame</Source><SourceDirection>+Z</SourceDirection><FeatureName></FeatureName></PrimaryAxis><SecondaryAxis><DefinedDirection>+Y</DefinedDirection><Source>ReferenceFrame</Source><SourceDirection>+X</SourceDirection><FeatureName></FeatureName></SecondaryAxis></Value></Frame><Frame><Id>Frame5</Id><Value><Name>BotH</Name><Origin><Source>GeometricFeature</Source><FeatureName>circular curve 175</FeatureName></Origin><PrimaryAxis><DefinedDirection>+X</DefinedDirection><Source>ReferenceFrame</Source><SourceDirection>+Z</SourceDirection><FeatureName></FeatureName></PrimaryAxis><SecondaryAxis><DefinedDirection>+Y</DefinedDirection><Source>ReferenceFrame</Source><SourceDirection>+X</SourceDirection><FeatureName></FeatureName></SecondaryAxis></Value></Frame><Frame><Id>Frame6</Id><Value><Name>Measure</Name><Origin><Source>GeometricFeature</Source><FeatureName>circular curve 101</FeatureName></Origin><PrimaryAxis><DefinedDirection>+Z</DefinedDirection><Source>ReferenceFrame</Source><SourceDirection>+Y</SourceDirection><FeatureName></FeatureName></PrimaryAxis><SecondaryAxis><DefinedDirection>+X</DefinedDirection><Source>ReferenceFrame</Source><SourceDirection>+Z</SourceDirection><FeatureName></FeatureName></SecondaryAxis></Value></Frame></Frames>  GraphicType=FromGeometry  MarkerShape=Sphere  MarkerSize=10  GraphicVisPropType=SimpleVisualProperties  GraphicDiffuseColor=[0.4 0.4 0.4]  GraphicSpecularColor=[0.5 0.5 0.5 1.0]  GraphicAmbientColor=[0.15 0.15 0.15 1.0]  GraphicEmissiveColor=[0.0 0.0 0.0 1.0]  GraphicShininess=75  GraphicOpacity=smiData.Solid(10).opacity
  LB : PMIOPort  Side=Left
  TopH : PMIOPort  Port=2  Side=Left
  BotH : PMIOPort  Port=3  Side=Right
  MidH : PMIOPort  Port=4  Side=Right
  connections:
  LB/RConn1 -- Solid/LConn1
  MidH/RConn1 -- Solid/RConn2
  BotH/RConn1 -- Solid/LConn3
  TopH/RConn1 -- Solid/LConn2

== system sm_3d_printer/3D Printer/Gantry Assembly/Guide Rail B ==
  Solid : sm_lib/Body Elements/File Solid  ExtGeomFileName=Guide_Rail_y.STEP  UnitType=FromFile  ExtGeomFileUnits=m  StepReaderType=HEX  ExportConvexHullGeometry=off  InertiaType=Custom  Mass=smiData.Solid(1).mass  MassUnits=kg  CenterOfMass=smiData.Solid(1).CoM  CenterOfMassUnits=m  MomentsOfInertia=smiData.Solid(1).MoI  MomentsOfInertiaUnits=kg*m^2  ProductsOfInertia=smiData.Solid(1).PoI  ProductsOfInertiaUnits=kg*m^2  BasedOnType=DensityFromFile  Density=1000  DensityUnits=kg/m^3  DoExposeReferenceFrame=off  SerializedFrames=<Frames><Frame><Id>Frame1</Id><Value><Name>LS</Name><Origin><Source>GeometricFeature</Source><FeatureName>circular curve 3</FeatureName></Origin><PrimaryAxis><DefinedDirection>+X</DefinedDirection><Source>ReferenceFrame</Source><SourceDirection>+Z</SourceDirection><FeatureName></FeatureName></PrimaryAxis><SecondaryAxis><DefinedDirection>+Y</DefinedDirection><Source>ReferenceFrame</Source><SourceDirection>+X</SourceDirection><FeatureName></FeatureName></SecondaryAxis></Value></Frame><Frame><Id>Frame2</Id><Value><Name>RS</Name><Origin><Source>GeometricFeature</Source><FeatureName>circular curve 4</FeatureName></Origin><PrimaryAxis><DefinedDirection>+X</DefinedDirection><Source>ReferenceFrame</Source><SourceDirection>+Z</SourceDirection><FeatureName></FeatureName></PrimaryAxis><SecondaryAxis><DefinedDirection>+Y</DefinedDirection><Source>ReferenceFrame</Source><SourceDirection>+X</SourceDirection><FeatureName></FeatureName></SecondaryAxis></Value></Frame></Frames>  GraphicType=FromGeometry  MarkerShape=Sphere  MarkerSize=10  GraphicVisPropType=SimpleVisualProperties  GraphicDiffuseColor=smiData.Solid(1).color  GraphicSpecularColor=[0.5 0.5 0.5 1.0]  GraphicAmbientColor=[0.15 0.15 0.15 1.0]  GraphicEmissiveColor=[0.0 0.0 0.0 1.0]  GraphicShininess=75  GraphicOpacity=smiData.Solid(1).opacity
  R : PMIOPort  Side=Right
  L : PMIOPort  Port=2  Side=Left
  connections:
  Solid/LConn1 -- L/RConn1
  Solid/RConn1 -- R/RConn1

== system sm_3d_printer/3D Printer/Gantry Assembly/Guide Rail T ==
  Solid : sm_lib/Body Elements/File Solid  ExtGeomFileName=Guide_Rail_y.STEP  UnitType=FromFile  ExtGeomFileUnits=m  StepReaderType=HEX  ExportConvexHullGeometry=off  InertiaType=Custom  Mass=smiData.Solid(1).mass  MassUnits=kg  CenterOfMass=smiData.Solid(1).CoM  CenterOfMassUnits=m  MomentsOfInertia=smiData.Solid(1).MoI  MomentsOfInertiaUnits=kg*m^2  ProductsOfInertia=smiData.Solid(1).PoI  ProductsOfInertiaUnits=kg*m^2  BasedOnType=Density  Density=2700  DensityUnits=kg/m^3  DoExposeReferenceFrame=off  SerializedFrames=<Frames><Frame><Id>Frame1</Id><Value><Name>LS</Name><Origin><Source>GeometricFeature</Source><FeatureName>circular curve 3</FeatureName></Origin><PrimaryAxis><DefinedDirection>+X</DefinedDirection><Source>ReferenceFrame</Source><SourceDirection>+Z</SourceDirection><FeatureName></FeatureName></PrimaryAxis><SecondaryAxis><DefinedDirection>+Y</DefinedDirection><Source>ReferenceFrame</Source><SourceDirection>+X</SourceDirection><FeatureName></FeatureName></SecondaryAxis></Value></Frame><Frame><Id>Frame2</Id><Value><Name>RS</Name><Origin><Source>GeometricFeature</Source><FeatureName>circular curve 4</FeatureName></Origin><PrimaryAxis><DefinedDirection>+X</DefinedDirection><Source>ReferenceFrame</Source><SourceDirection>+Z</SourceDirection><FeatureName></FeatureName></PrimaryAxis><SecondaryAxis><DefinedDirection>+Y</DefinedDirection><Source>ReferenceFrame</Source><SourceDirection>+X</SourceDirection><FeatureName></FeatureName></SecondaryAxis></Value></Frame></Frames>  GraphicType=FromGeometry  MarkerShape=Sphere  MarkerSize=10  GraphicVisPropType=SimpleVisualProperties  GraphicDiffuseColor=smiData.Solid(1).color  GraphicSpecularColor=[0.5 0.5 0.5 1.0]  GraphicAmbientColor=[0.15 0.15 0.15 1.0]  GraphicEmissiveColor=[0.0 0.0 0.0 1.0]  GraphicShininess=75  GraphicOpacity=smiData.Solid(1).opacity
  R : PMIOPort  Side=Right
  L : PMIOPort  Port=2  Side=Left
  connections:
  Solid/LConn1 -- L/RConn1
  Solid/RConn1 -- R/RConn1

== system sm_3d_printer/3D Printer/Gantry Assembly/Lead Screw ==
  Solid : sm_lib/Body Elements/File Solid  ExtGeomFileName=Screw_y.STEP  UnitType=FromFile  ExtGeomFileUnits=m  StepReaderType=HEX  ExportConvexHullGeometry=off  InertiaType=Custom  Mass=smiData.Solid(12).mass  MassUnits=kg  CenterOfMass=smiData.Solid(12).CoM  CenterOfMassUnits=m  MomentsOfInertia=smiData.Solid(12).MoI  MomentsOfInertiaUnits=kg*m^2  ProductsOfInertia=smiData.Solid(12).PoI  ProductsOfInertiaUnits=kg*m^2  BasedOnType=Density  Density=2700  DensityUnits=kg/m^3  DoExposeReferenceFrame=off  SerializedFrames=<Frames><Frame><Id>Frame1</Id><Value><Name>L</Name><Origin><Source>GeometricFeature</Source><FeatureName>planar surface 1</FeatureName></Origin><PrimaryAxis><DefinedDirection>+X</DefinedDirection><Source>ReferenceFrame</Source><SourceDirection>+X</SourceDirection><FeatureName></FeatureName></PrimaryAxis><SecondaryAxis><DefinedDirection>+Z</DefinedDirection><Source>ReferenceFrame</Source><SourceDirection>+Z</SourceDirection><FeatureName></FeatureName></SecondaryAxis></Value></Frame><Frame><Id>Frame2</Id><Value><Name>R</Name><Origin><Source>GeometricFeature</Source><FeatureName>circular curve 4</FeatureName></Origin><PrimaryAxis><DefinedDirection>+X</DefinedDirection><Source>ReferenceFrame</Source><SourceDirection>+X</SourceDirection><FeatureName></FeatureName></PrimaryAxis><SecondaryAxis><DefinedDirection>+Z</DefinedDirection><Source>ReferenceFrame</Source><SourceDirection>+Z</SourceDirection><FeatureName></FeatureName></SecondaryAxis></Value></Frame></Frames>  GraphicType=FromGeometry  MarkerShape=Sphere  MarkerSize=10  GraphicVisPropType=SimpleVisualProperties  GraphicDiffuseColor=[0.6 0.6 0.6]  GraphicSpecularColor=[0.5 0.5 0.5 1.0]  GraphicAmbientColor=[0.15 0.15 0.15 1.0]  GraphicEmissiveColor=[0.0 0.0 0.0 1.0]  GraphicShininess=75  GraphicOpacity=smiData.Solid(1).opacity
  L : PMIOPort  Side=Right
  R : PMIOPort  Port=2  Side=Left
  connections:
  R/RConn1 -- Solid/RConn1
  L/RConn1 -- Solid/LConn1
